simulink model "H8_LPV"  (R2022a)
settings: Solver=VariableStepAuto  StartTime=0.0  StopTime=50  RelTol=1e-3
values from neighbouring files (symbols this model uses):
  K1 = double(Y1)*inv(double(X))    [H8_LPV_controller.m]    (also in H8_robust_stateflow.m = H8_robust_f( Ag1,Ag2,Bg1,Bg2,Eg1,Eg2,Cg1,Cg2,Dg1,Dg2,Fg1,Fg2)
  K2 = double(Y1)*inv(double(X))    [H8_LPV_controller.m]    (also in H8_robust_stateflow.m = H8_robust_f( Ag1,Ag2,Bg1,Bg2,Eg1,Eg2,Cg1,Cg2,Dg1,Dg2,Fg1,Fg2)
  Kc = 938    [H2.m]    (also in H2_alpha.m; H8_Alpha.m; H8_LPV_controller.m; H8_robust_mass.m)
  ks = 27000    [H2.m]    (also in H2_alpha.m; H8_Alpha.m; H8_LPV_controller.m; H8_robust_mass.m)
  ku = 228000    [H2.m]    (also in H2_alpha.m; H8_Alpha.m; H8_LPV_controller.m; H8_robust_mass.m)
  mu = 35.5    [H2.m]    (also in H2_alpha.m; H8_Alpha.m; H8_LPV_controller.m; H8_robust_mass.m)
undefined symbols (not defined in the file or in its folder): Ad, Az, Bd, Bz, Cd, Cz, Dd, Dz, sigbuilder_block
libraries: simulink x1
settings Model: Creator=User  LastModifiedBy=User

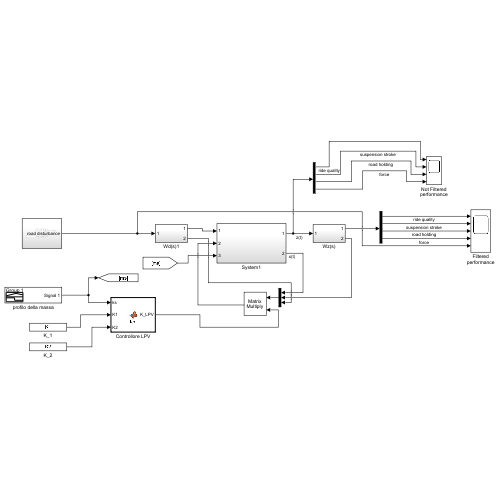
[thumbnail: Simulink's stored preview of the top-level diagram]
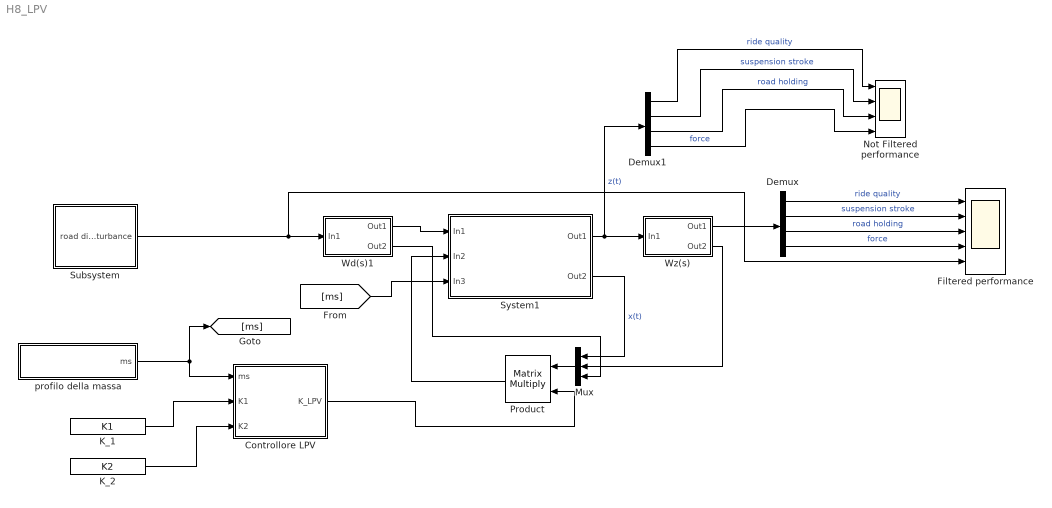
== system H8_LPV ==
  Controllore LPV : MATLAB Function  TreatAsAtomicUnit=on
  Demux : Demux
  Demux1 : Demux
  Filtered performance : Scope  NumInputPorts=5
  K_1 : Constant  Value=K1
  K_2 : Constant  Value=K2
  Mux : Mux  Inputs=3
  Not Filtered performance : Scope  NumInputPorts=4
  Product : Product  Multiplication=Matrix(*)
  Subsystem : Subsystem
  System1 : Subsystem
  Wd(s)1 : Subsystem
  Wz(s) : Subsystem
  profilo della massa : Subsystem  Tag=STV Subsys  LoadFcn=sigbuilder_block('load');  StartFcn=sigbuilder_block('start');  StopFcn=sigbuilder_block('stop');  ClipboardFcn=sigbuilder_block('clipboard');  mask(Sigbuilder block){tuvar=[0:10]}
      mask help: Simulink:masks:SigbuilderBlock_MD
      mask init:
      | if ~strcmp(get_param(bdroot(gcbh),'SimulationStatus'),'stopped') tuvar = sigbuilder_block('maskInit'); end
      settings: CopyFcn=sigbuilder_block('copy');  DeleteFcn=sigbuilder_block('delete');  ModelCloseFcn=sigbuilder_block('modelClose');  PreSaveFcn=sigbuilder_block('preSave');  PauseFcn=sigbuilder_block('pause');  ContinueFcn=sigbuilder_block('continue');  NameChangeFcn=sigbuilder_block('namechange');  OpenFcn=sigbuilder_block('open',[5.4 12 1141.2 574.2 ]);  CloseFcn=sigbuilder_block('close');
      mask Display: plot(0, 0, 100, 100,[2, 2, 32, 32, 2], [68, 8, 8, 68, 68],[32, 2], [38, 38], [32, 19, 2],[53, 60, 44], [32, 17, 17, 2],[16, 16, 31, 31]);txt = getActiveGroup(gcbh);text(2, 100, txt,'verticalAlignment', 'top');
  wires:
  Wz(s)/2(Out2) -> Mux/2
  Wz(s)/1(Out1) -> Demux/1
  Demux/1 -> Filtered performance/1  "ride quality"
  System1/1(Out1) -> Demux1/1, Wz(s)/1(In1)  "z(t)"
  Product/1 -> System1/2(In2)
  Demux/2 -> Filtered performance/2  "suspension stroke"
  Mux/1 -> Product/1
  System1/2(Out2) -> Mux/1  "x(t)"
  Wd(s)1/1(Out1) -> System1/1(In1)
  Wd(s)1/2(Out2) -> Mux/3
  Demux/3 -> Filtered performance/3  "road holding"
  Demux1/1 -> Not Filtered performance/1  "ride quality"
  Demux1/2 -> Not Filtered performance/2  "suspension stroke"
  Demux1/3 -> Not Filtered performance/3  "road holding"
  Demux/4 -> Filtered performance/4  "force"
  Demux1/4 -> Not Filtered performance/4  "force"
  profilo della massa/1(ms) -> [ms], Controllore LPV/1(ms)
  K_2/1 -> Controllore LPV/3(K2)
  K_1/1 -> Controllore LPV/2(K1)
  Subsystem/1(road disturbance) -> Filtered performance/5, Wd(s)1/1(In1)
  Controllore LPV/1(K_LPV) -> Product/2
  [ms] -> System1/3(In3)

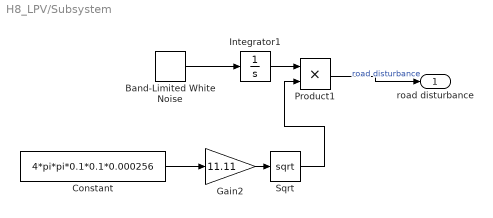
== system H8_LPV/Subsystem ==
  Band-Limited White Noise : simulink/Sources/Band-Limited White Noise  Cov=[0.1]  Ts=0.1  seed=[23341]
  Constant : Constant  Value=4*pi*pi*0.1*0.1*0.000256
  Gain2 : Gain  Gain=11.11
  Integrator1 : Integrator
  Product1 : Product
  Sqrt : Sqrt
  road disturbance : Outport
  wires:
  Band-Limited White Noise/1 -> Integrator1/1
  Gain2/1 -> Sqrt/1
  Constant/1 -> Gain2/1
  Integrator1/1 -> Product1/1
  Sqrt/1 -> Product1/2
  Product1/1 -> road disturbance/1  "road disturbance"

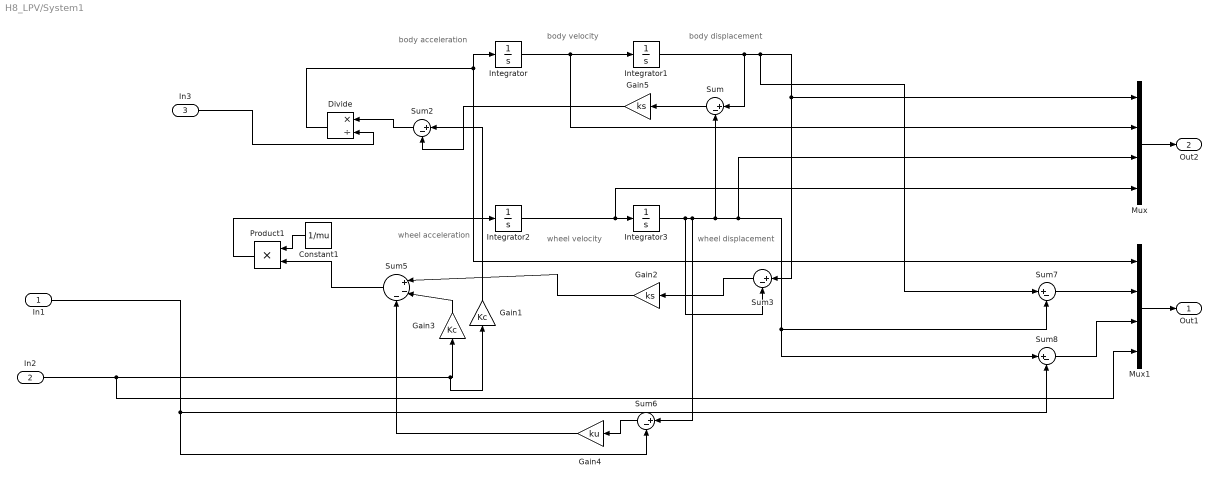
== system H8_LPV/System1 ==
  note: body acceleration
  note: wheel velocity
  note: wheel displacement
  note: body velocity
  note: wheel acceleration
  note: body displacement
  In1 : Inport
  In2 : Inport  Port=2
  In3 : Inport  Port=3
  Constant1 : Constant  Value=1/mu
  Divide : Product  Inputs=*/
  Gain1 : Gain  Gain=Kc
  Gain2 : Gain  Gain=ks
  Gain3 : Gain  Gain=Kc
  Gain4 : Gain  Gain=ku
  Gain5 : Gain  Gain=ks
  Integrator{,1..3} (4 alike) : Integrator
  Mux : Mux
  Mux1 : Mux
  Product1 : Product
  Sum{,2..3,6..8} (6 alike) : Sum  Inputs=|+-
  Sum5 : Sum  Inputs=|+--
  Out1 : Outport
  Out2 : Outport  Port=2
  wires:
  Sum8/1 -> Mux1/3
  Sum7/1 -> Mux1/2
  Integrator/1 -> Mux/2, Integrator1/1
  Sum6/1 -> Gain4/1
  In1/1 -> Sum8/2, Sum6/2
  Integrator1/1 -> Sum7/1, Sum3/1, Mux/1, Sum/1
  Divide/1 -> Integrator/1, Mux1/1
  Gain5/1 -> Sum2/2
  Gain2/1 -> Sum5/1
  Sum/1 -> Gain5/1
  Integrator3/1 -> Mux/3, Sum8/1, Sum7/2, Sum/2, Sum6/1, Sum3/2
  Integrator2/1 -> Mux/4, Integrator3/1
  Sum3/1 -> Gain2/1
  Gain4/1 -> Sum5/3
  In2/1 -> Mux1/4, Gain1/1, Gain3/1
  Mux/1 -> Out2/1
  Mux1/1 -> Out1/1
  Gain1/1 -> Sum2/1
  Constant1/1 -> Product1/1
  Sum5/1 -> Product1/2
  Product1/1 -> Integrator2/1
  Gain3/1 -> Sum5/2
  In3/1 -> Divide/2
  Sum2/1 -> Divide/1

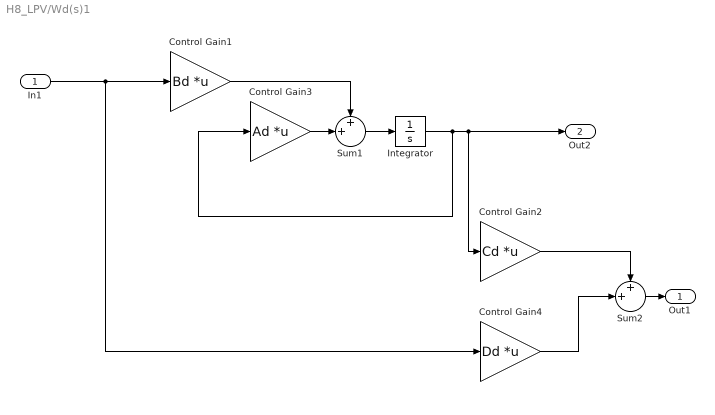
== system H8_LPV/Wd(s)1 ==
  In1 : Inport
  Control Gain1 : Gain  Gain=Bd  Multiplication=Matrix(K*u)
  Control Gain2 : Gain  Gain=Cd  Multiplication=Matrix(K*u)
  Control Gain3 : Gain  Gain=Ad  Multiplication=Matrix(K*u)
  Control Gain4 : Gain  Gain=Dd  Multiplication=Matrix(K*u)
  Integrator : Integrator
  Sum1 : Sum  Inputs=++|
  Sum2 : Sum  Inputs=++|
  Out1 : Outport
  Out2 : Outport  Port=2
  wires:
  In1/1 -> Control Gain4/1, Control Gain1/1
  Integrator/1 -> Control Gain2/1, Out2/1, Control Gain3/1
  Sum1/1 -> Integrator/1
  Control Gain1/1 -> Sum1/1
  Control Gain3/1 -> Sum1/2
  Sum2/1 -> Out1/1
  Control Gain2/1 -> Sum2/1
  Control Gain4/1 -> Sum2/2

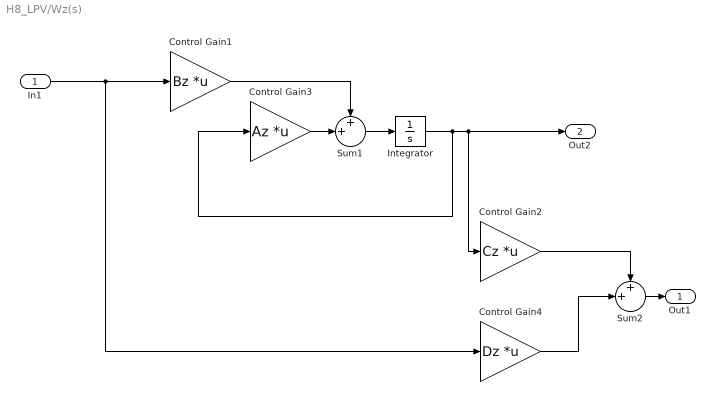
== system H8_LPV/Wz(s) ==
  In1 : Inport
  Control Gain1 : Gain  Gain=Bz  Multiplication=Matrix(K*u)
  Control Gain2 : Gain  Gain=Cz  Multiplication=Matrix(K*u)
  Control Gain3 : Gain  Gain=Az  Multiplication=Matrix(K*u)
  Control Gain4 : Gain  Gain=Dz  Multiplication=Matrix(K*u)
  Integrator : Integrator
  Sum1 : Sum  Inputs=++|
  Sum2 : Sum  Inputs=++|
  Out1 : Outport
  Out2 : Outport  Port=2
  wires:
  In1/1 -> Control Gain4/1, Control Gain1/1
  Integrator/1 -> Control Gain2/1, Out2/1, Control Gain3/1
  Sum1/1 -> Integrator/1
  Control Gain1/1 -> Sum1/1
  Control Gain3/1 -> Sum1/2
  Sum2/1 -> Out1/1
  Control Gain2/1 -> Sum2/1
  Control Gain4/1 -> Sum2/2

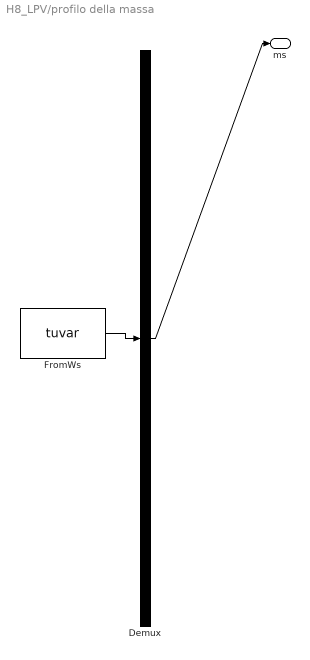
== system H8_LPV/profilo della massa ==
  Demux : Demux  Tag=STV Demux  Outputs=1
      settings: DisplayOption=none
  FromWs : FromWorkspace  Tag=STV FromWs  VariableName=tuvar
      SigBuilderData=|
      | common.afterFinalStr = 'Extrapolate'
      | common.sampleTime = 0
      | dataSet.timeRange = [0 55]
      | dataSet.name = 'Group 1'
      | sbobj.Groups.Name = 'Group 1'
      | sbobj.Groups.Signals.Name = 'ms'
      | sbobj.Groups.Signals.XData = [0 10 10 20 20 30 30 40 40 49.95 49.95 55]
      | sbobj.Groups.Signals.YData = [200 201 273 275 240 240 289 289 315 315 401 400]
      | sbobj.Groups.TimeRange = [0 55]
  ms : Outport  Tag=STV Outport
  wires:
  FromWs/1 -> Demux/1
  Demux/1 -> ms/1

== matlab function H8_LPV/Controllore LPV ==
  data: ms input; K_LPV output; K1 input; K2 input
function K_LPV = fcn(ms, K1, K2 )
    msmin=200;
    msmax=400;
    p= ( ms - msmin ) / (msmax - msmin);
    K_LPV= p * K1 + (1- p) *K2;
    
end
